simulink model "PMSM_sfunction"  (R2014b)
settings: Solver=ode23t  StartTime=0.0  StopTime=0.1  RelTol=1e-3
InitFcn:
  | Ts=50e-6;
  | Ld = 8.5e-3;
  | R = 2.875;
libraries: powerlib_extras x3, powerlib x1
settings Model: CovSFcnEnable=on  Creator=Administrator  LastModifiedBy=Lei
settings DataIOCC: SignalLoggingSaveFormat=ModelDataLogs
settings OptimizationCC: ExpressionDepthLimit=2147483647  InitFltsAndDblsToZero=on
settings DebuggingCC: SaveWithParameterizedLinksMsg=none  UnderspecifiedInitializationDetection=Classic  MergeDetectMultiDrivingBlocksExec=none  FcnCallInpInsideContextMsg=UseLocalSettings  FrameProcessingCompatibilityMsg=error  StateNameClashWarn=warning
settings GRTTargetCC: TargetFcnLib=ansi_tfl_tmw.mat  CombineOutputUpdateFcns=off  GRTInterface=on

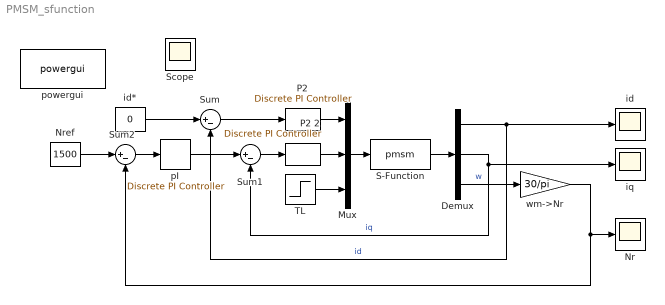
== system PMSM_sfunction ==
  Demux : Demux  Outputs=3
  Mux : Mux  Inputs=3
  Nr : Scope
      settings: SaveName=Nr
  Nref : Constant  Value=1500
  "P2 " : powerlib_extras/Discrete  Control Blocks/Discrete PI Controller  Kp=Ld*2100  Ki=R*2100  Par_Limits=[250 -250]  Init=0  Ts=Ts
  P2 2 : powerlib_extras/Discrete  Control Blocks/Discrete PI Controller  Kp=Ld*2100  Ki=R*2100  Par_Limits=[250 -250]  Init=0  Ts=Ts
  S-Function : S-Function  FunctionName=pmsm  EnableBusSupport=off
  Sum : Sum  Inputs=|+-
  Sum1 : Sum  Inputs=|+-
  Sum2 : Sum  Inputs=|+-
  TL : Step  Time=0.05  After=10  SampleTime=0
  id : Scope
      settings: SaveName=Id
  id* : Constant  Value=0
  iq : Scope
      settings: SaveName=Iq
  "pI " : powerlib_extras/Discrete  Control Blocks/Discrete PI Controller  Kp=0.06  Ki=10  Par_Limits=[300 -300]  Init=0  Ts=Ts
  powergui : powerlib/powergui  SimulationMode=Continuous  SolverType=Tustin/Backward Euler (TBE)  SampleTime=50e-6  frequency=60  SPID=off  DisableSnubberDevices=off  DisableRonSwitches=off  DisableVfSwitches=off  SwTol=0  DisplayEquations=off  Interpol=off  methode=off  Ts=0  frequencyindice=0  Pbase=100e6  ErrMax=1e-4  Iterations=50  UnitsV=kV  UnitsW=MW  FunctionMessages=off  echomessages=off  HookPort=off  EnableUseOfTLC=off  x0status=blocks  RestoreLinks=warning  ResistiveCurrentMeasurement=off  Frange=[0:2:500]  Ylog=off  Xlog=on  ShowGrid=off  save=off  variable=ZData  structure=0  ZoomFFT=off  StartTime=0.0  cycles=1  DisplayStyle=1  fundamental=60  FreqAxis=off  MaxFrequency=1000  frequencyindicesteady=1  RmsSteady=1  display=off
  wm->Nr : Gain  Gain=30/pi
  Scope : Scope
  wires:
  Sum1/1 -> P2 2/1
  "pI "/1 -> Sum1/1
  Sum2/1 -> "pI "/1
  wm->Nr/1 -> Nr/1, Sum2/2
  Nref/1 -> Sum2/1
  Demux/1 -> id/1, Sum/2  "id"
  Demux/2 -> iq/1, Sum1/2  "iq"
  P2 2/1 -> Mux/2
  "P2 "/1 -> Mux/1
  Demux/3 -> wm->Nr/1  "w"
  TL/1 -> Mux/3
  Mux/1 -> S-Function/1
  S-Function/1 -> Demux/1
  Sum/1 -> "P2 "/1
  id*/1 -> Sum/1
